simulink model "HDLPayloadFull"  (R2024a)
settings: Solver=FixedStepDiscrete  StartTime=0.0  StopTime=stopTime  RelTol=1e-3
values from neighbouring files (symbols this model uses):
  pWords = [pWords binl2str(pBitsRaw{i})]    [testPayloadFull.m]
undefined symbols (not defined in the file or in its folder): CONST, msgIn
libraries: dspsrcs4 x8, simulink x2, hdlsllib x2, whdlutilities x1, HDL_ieee_8021513 x1
settings Model: DataTypeOverride=Off  SimulationMode=accelerator  Creator=cotti  LastModifiedBy=cotti
settings OptimizationCC: BlockReduction=off  ConditionallyExecuteInputs=off  DefaultParameterBehavior=Inlined  InheritOutputTypeSmallerThanSingle=on
settings DebuggingCC: AlgebraicLoopMsg=error  ArtificialAlgebraicLoopMsg=error  SingleTaskRateTransMsg=error  UnconnectedInputMsg=warning  UnconnectedOutputMsg=warning  UnconnectedLineMsg=warning
settings HardwareCC: ProdBitPerPointer=32  ProdBitPerSizeT=32  ProdBitPerPtrDiffT=32  ProdLargestAtomicFloat=None  ProdIntDivRoundTo=Undefined  ProdEndianess=Unspecified  ProdWordSize=32  ProdHWDeviceType=ASIC/FPGA->ASIC/FPGA  TargetBitPerLong=64  TargetBitPerPointer=64  TargetBitPerSizeT=64  TargetBitPerPtrDiffT=64  TargetLongLongMode=on  TargetIntDivRoundTo=Zero  TargetEndianess=LittleEndian  TargetWordSize=64  TargetHWDeviceType=Custom Processor->MATLAB Host Computer  ProdEqTarget=off

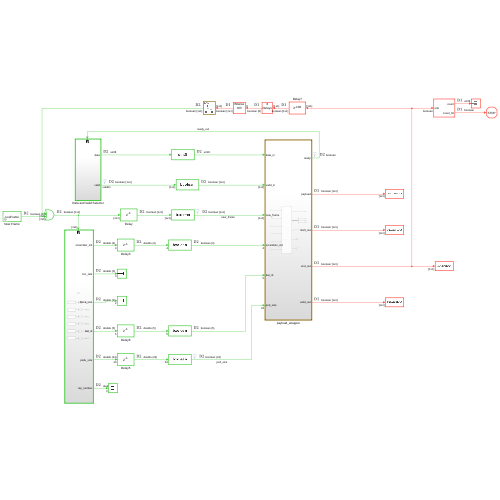
[thumbnail: Simulink's stored preview of the top-level diagram]
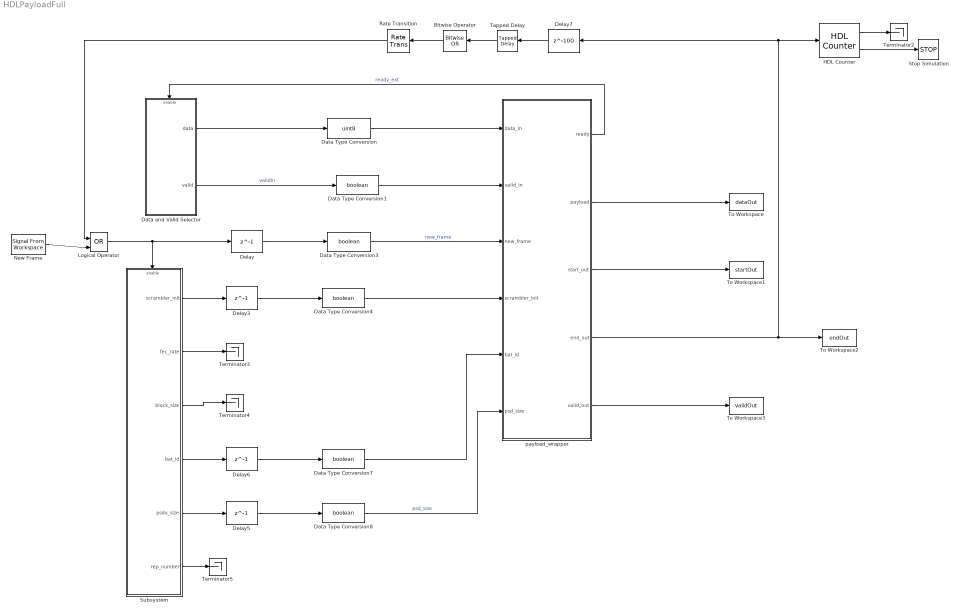
== system HDLPayloadFull ==
  Bitwise Operator : simulink/Logic and Bit Operations/Bitwise Operator  logicop=OR  UseBitMask=off  BitMask=bin2dec('11011001')  BitMaskRealWorld=Stored Integer
      settings: LibrarySourceBlock=|
      | hdlsllib/Logic and Bit
      | Operations/Bitwise
      | Operator
  Data Type Conversion : DataTypeConversion  OutDataTypeStr=uint8  SaturateOnIntegerOverflow=off  RndMeth=Floor
  Data Type Conversion{1,3..4,7..8} (5 alike) : DataTypeConversion  OutDataTypeStr=boolean  SaturateOnIntegerOverflow=off  RndMeth=Floor
  Data and Valid Selector : Subsystem  TreatAsAtomicUnit=on
  Delay{,3,5..6} (4 alike) : Delay  DelayLength=1  InitialCondition=0  UseCircularBuffer=on
  Delay7 : Delay  DelayLength=100  InitialCondition=0  UseCircularBuffer=on
  HDL Counter : hdlsllib/Sources/HDL Counter  CountType=Count limited  CountInit=0  CountStep=1  CountMax=length(msgIn)  CountFromType=Initial value  CountFrom=0  CountResetPort=off  CountLoadPort=off  CountEnbPort=on  CountDirPort=off  CountHitOutputPort=on  CountDataType=Unsigned  CountWordLen=8  CountFracLen=0  CountSampTime=1
  Logical Operator : Logic  Operator=OR  IconShape=distinctive  AllPortsSameDT=off  OutDataTypeStr=boolean
  New Frame : dspsrcs4/Signal From Workspace  X=newFrame  Ts=8/CONST.fs  nsamps=1  OutputAfterFinalValue=Setting to zero  ignoreOrWarnInputAndFrameLengths=off  OutputFrames=off
  Rate Transition : RateTransition  OutPortSampleTimeOpt=Multiple of input port sample time  OutPortSampleTimeMultiple=8
  Stop Simulation : Stop
  Subsystem : Subsystem
  Tapped Delay : simulink/Discrete/Tapped Delay  vinit=0.0  samptime=-1  NumDelays=8  DelayOrder=Oldest  includeCurrent=off
      settings: LibrarySourceBlock=hdlsllib/Discrete/Tapped Delay
  Terminator{2..5} (4 alike) : Terminator
  To Workspace : ToWorkspace  VariableName=dataOut  SampleTime=1/CONST.fs
      settings: Save2DSignal=2-D array (concatenate along first dimension)
  To Workspace1 : ToWorkspace  VariableName=startOut  SampleTime=1/CONST.fs
      settings: Save2DSignal=2-D array (concatenate along first dimension)
  To Workspace2 : ToWorkspace  VariableName=endOut  SampleTime=1/CONST.fs
      settings: Save2DSignal=2-D array (concatenate along first dimension)
  To Workspace3 : ToWorkspace  VariableName=validOut  SampleTime=1/CONST.fs
      settings: Save2DSignal=2-D array (concatenate along first dimension)
  payload_wrapper : Subsystem  TreatAsAtomicUnit=on
  wires:
  payload_wrapper/3(start_out) -> To Workspace1/1
  payload_wrapper/5(valid_out) -> To Workspace3/1
  payload_wrapper/4(end_out) -> HDL Counter/1, Delay7/1, To Workspace2/1
  Delay5/1 -> Data Type Conversion8/1
  Delay3/1 -> Data Type Conversion4/1
  Delay/1 -> Data Type Conversion3/1
  Data and Valid Selector/2(valid) -> Data Type Conversion1/1  "validIn"
  Delay6/1 -> Data Type Conversion7/1
  Data and Valid Selector/1(data) -> Data Type Conversion/1
  HDL Counter/2 -> Stop Simulation/1
  HDL Counter/1 -> Terminator2/1
  Logical Operator/1 -> Subsystem/Enable, Delay/1
  New Frame/1 -> Logical Operator/2
  Bitwise Operator/1 -> Rate Transition/1
  Rate Transition/1 -> Logical Operator/1
  Tapped Delay/1 -> Bitwise Operator/1
  Subsystem/1(scrambler_init) -> Delay3/1
  Subsystem/4(bat_id) -> Delay6/1
  Subsystem/5(psdu_size) -> Delay5/1
  Delay7/1 -> Tapped Delay/1
  Subsystem/2(fec_rate) -> Terminator3/1
  Subsystem/3(block_size) -> Terminator4/1
  Subsystem/6(rep_number) -> Terminator5/1
  Data Type Conversion/1 -> payload_wrapper/1(data_in)
  Data Type Conversion1/1 -> payload_wrapper/2(valid_in)
  Data Type Conversion3/1 -> payload_wrapper/3(new_frame)  "new_frame"
  Data Type Conversion4/1 -> payload_wrapper/4(scrambler_init)
  Data Type Conversion7/1 -> payload_wrapper/5(bat_id)
  Data Type Conversion8/1 -> payload_wrapper/6(psd_size)  "psd_size"
  payload_wrapper/1(ready) -> Data and Valid Selector/Enable  "ready_ext"
  payload_wrapper/2(payload) -> To Workspace/1

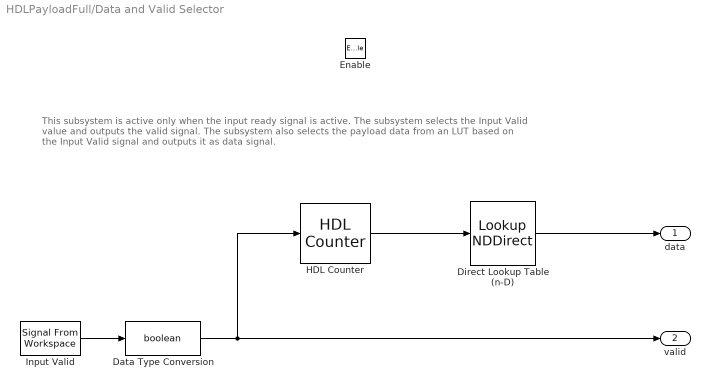
== system HDLPayloadFull/Data and Valid Selector ==
  note: This subsystem is active only when the input ready signal is active. The subsystem selects the Input Valid value and outputs the valid signal.
      | The subsystem also selects the payload data from an LUT based on the Input Valid signal and outputs it as data signal.
  Enable : EnablePort
  Data Type Conversion : DataTypeConversion  OutDataTypeStr=boolean  SaturateOnIntegerOverflow=off  RndMeth=Floor
  Direct Lookup Table (n-D) : LookupNDDirect  NumberOfTableDimensions=1  Table=uint8(pWords')  DiagnosticForOutOfRangeInput=Error  TableDataTypeStr=uint8
  HDL Counter : hdlsllib/Sources/HDL Counter  CountType=Count limited  CountInit=0  CountStep=1  CountMax=length(pWords) -1  CountFromType=Initial value  CountFrom=0  CountResetPort=off  CountLoadPort=off  CountEnbPort=on  CountDirPort=off  CountHitOutputPort=off  CountDataType=Unsigned  CountWordLen=nextpow2(length(pWords))  CountFracLen=0  CountSampTime=1
  Input Valid : dspsrcs4/Signal From Workspace  X=validIn  Ts=8/CONST.fs  nsamps=1  OutputAfterFinalValue=Setting to zero  ignoreOrWarnInputAndFrameLengths=off  OutputFrames=off
  data : Outport  InitialOutput=0  VectorParamsAs1DForOutWhenUnconnected=off
  valid : Outport  Port=2  InitialOutput=0  VectorParamsAs1DForOutWhenUnconnected=off
  wires:
  HDL Counter/1 -> Direct Lookup Table (n-D)/1
  Direct Lookup Table (n-D)/1 -> data/1
  Input Valid/1 -> Data Type Conversion/1
  Data Type Conversion/1 -> valid/1, HDL Counter/1

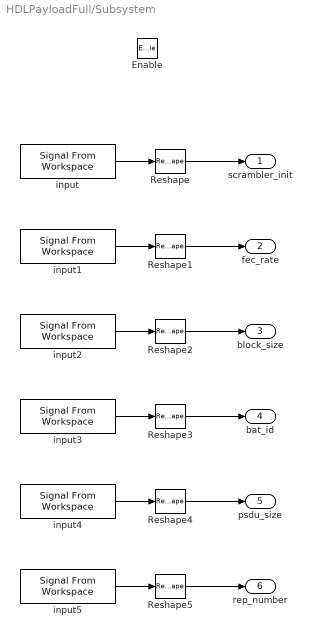
== system HDLPayloadFull/Subsystem ==
  Enable : EnablePort
  Reshape{,1..5} (6 alike) : Reshape
  input : dspsrcs4/Signal From Workspace  X=scramblerInitLSB  Ts=8/CONST.fs  nsamps=1  OutputAfterFinalValue=Setting to zero  ignoreOrWarnInputAndFrameLengths=off  OutputFrames=off
  input1 : dspsrcs4/Signal From Workspace  X=fecRateLSB  Ts=8/CONST.fs  nsamps=1  OutputAfterFinalValue=Setting to zero  ignoreOrWarnInputAndFrameLengths=off  OutputFrames=off
  input2 : dspsrcs4/Signal From Workspace  X=blockSizeLSB  Ts=8/CONST.fs  nsamps=1  OutputAfterFinalValue=Setting to zero  ignoreOrWarnInputAndFrameLengths=off  OutputFrames=off
  input3 : dspsrcs4/Signal From Workspace  X=batIdLSB  Ts=8/CONST.fs  nsamps=1  OutputAfterFinalValue=Setting to zero  ignoreOrWarnInputAndFrameLengths=off  OutputFrames=off
  input4 : dspsrcs4/Signal From Workspace  X=psduSizeLSB  Ts=8/CONST.fs  nsamps=1  OutputAfterFinalValue=Setting to zero  ignoreOrWarnInputAndFrameLengths=off  OutputFrames=off
  input5 : dspsrcs4/Signal From Workspace  X=repNumberLSB  Ts=8/CONST.fs  nsamps=1  OutputAfterFinalValue=Setting to zero  ignoreOrWarnInputAndFrameLengths=off  OutputFrames=off
  scrambler_init : Outport
  fec_rate : Outport  Port=2
  block_size : Outport  Port=3
  bat_id : Outport  Port=4
  psdu_size : Outport  Port=5
  rep_number : Outport  Port=6
  wires:
  input/1 -> Reshape/1
  input3/1 -> Reshape3/1
  input5/1 -> Reshape5/1
  input2/1 -> Reshape2/1
  input1/1 -> Reshape1/1
  input4/1 -> Reshape4/1
  Reshape/1 -> scrambler_init/1
  Reshape1/1 -> fec_rate/1
  Reshape2/1 -> block_size/1
  Reshape3/1 -> bat_id/1
  Reshape4/1 -> psdu_size/1
  Reshape5/1 -> rep_number/1

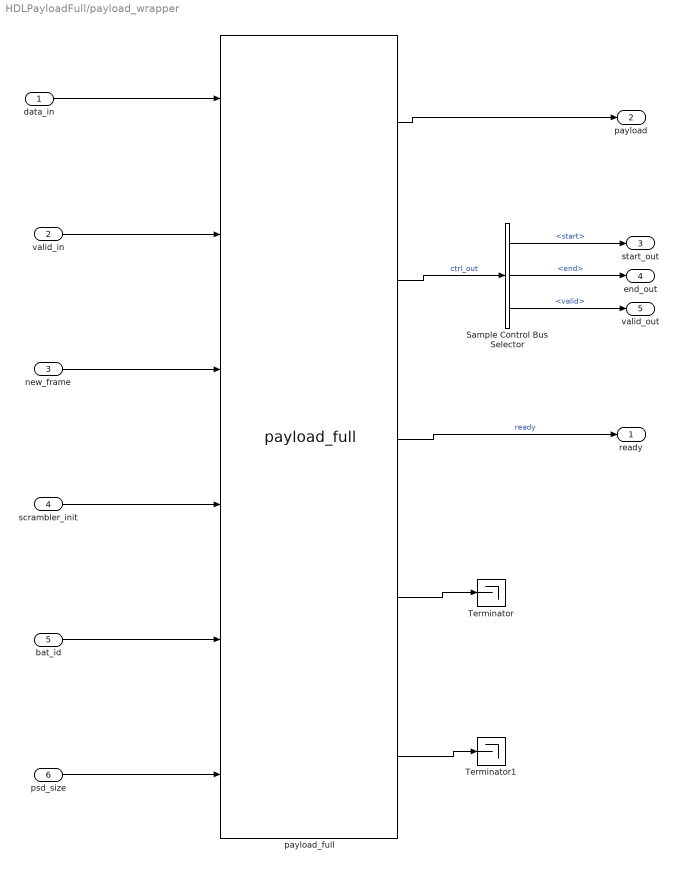
== system HDLPayloadFull/payload_wrapper ==
  data_in : Inport
  valid_in : Inport  Port=2
  new_frame : Inport  Port=3
  scrambler_init : Inport  Port=4
  bat_id : Inport  Port=5
  psd_size : Inport  Port=6
  Sample Control Bus Selector : whdlutilities/Sample Control Bus Selector  OutputSignals=start,end,valid
  Terminator : Terminator
  Terminator1 : Terminator
  payload_full : HDL_ieee_8021513/payload_full  SystemSampleTime=-1  VariantActivationTime=update diagram  AllowFlexibleInterface=on  Latency=0  AutoFrameSizeCalculation=off
      settings: SourceProductName=HDL IEEE 8021513
  ready : Outport
  payload : Outport  Port=2
  start_out : Outport  Port=3  VectorParamsAs1DForOutWhenUnconnected=off
  end_out : Outport  Port=4  VectorParamsAs1DForOutWhenUnconnected=off
  valid_out : Outport  Port=5  VectorParamsAs1DForOutWhenUnconnected=off
  wires:
  payload_full/1 -> payload/1
  psd_size/1 -> payload_full/6
  payload_full/4 -> Terminator/1
  payload_full/3 -> ready/1  "ready"
  data_in/1 -> payload_full/1
  bat_id/1 -> payload_full/5
  new_frame/1 -> payload_full/3
  scrambler_init/1 -> payload_full/4
  payload_full/5 -> Terminator1/1
  valid_in/1 -> payload_full/2
  payload_full/2 -> Sample Control Bus Selector/1  "ctrl_out"
  Sample Control Bus Selector/1 -> start_out/1  "<start>"
  Sample Control Bus Selector/2 -> end_out/1  "<end>"
  Sample Control Bus Selector/3 -> valid_out/1  "<valid>"
